simulink library "Differential_Gear1DShafts3Dfix"  (R2026a)
settings: Solver=VariableStepAuto
undefined symbols (not defined in the file): Shaft1D, Shaft3D, X, Y, Z
libraries: sm_lib x5, Differential_Components x2, fl_lib x2, nesl_utility x2, sdl_lib x1
Description:
  | Component of Simscape Vehicle Templates Library
  | 
  | Copyright 2018-2026 The MathWorks, Inc.
settings Model: Creator=smiller  LastModifiedBy=smiller

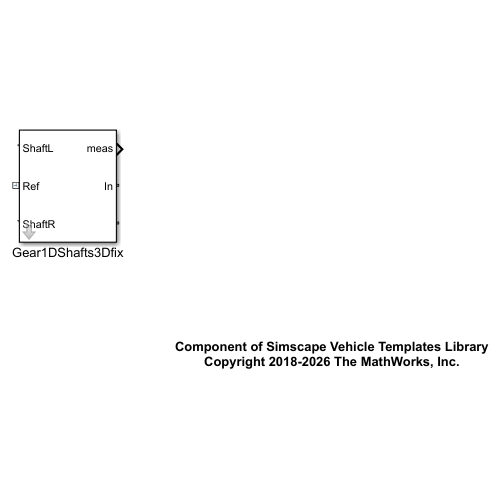
[thumbnail: Simulink's stored preview of the top-level diagram]
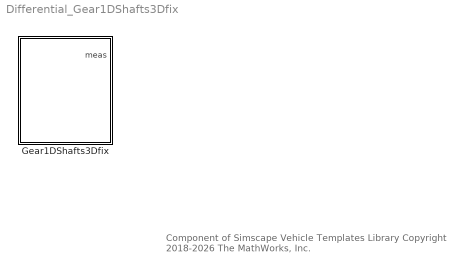
== system Differential_Gear1DShafts3Dfix ==
  note: Component of Simscape Vehicle Templates Library
      | Copyright 2018-2026 The MathWorks, Inc.
  Gear1DShafts3Dfix : Subsystem  VariantControl=Gear1DShafts3Dfix  mask(Differential 1D with static 3D Shafts){}
      mask help: Differential power transmission using 1D mechanical model. 3D shafts do not rotate and are included for 3D visualization and to contribute nonrotating mass and inertia.

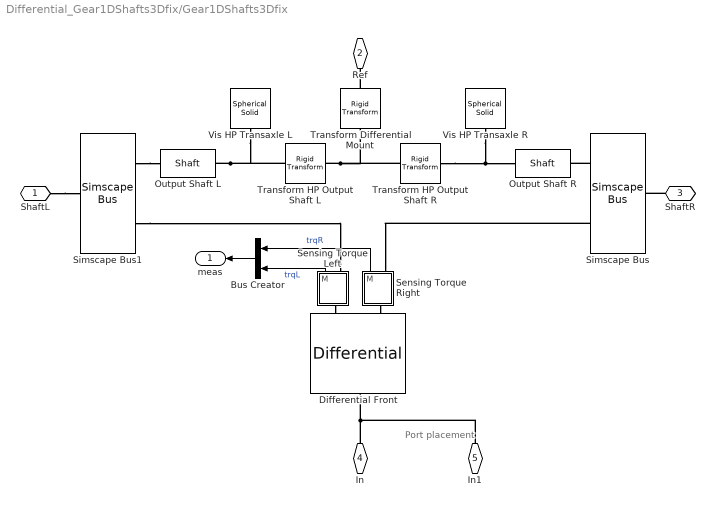
== system Differential_Gear1DShafts3Dfix/Gear1DShafts3Dfix ==
  note: Port
      | placement
  Bus Creator : BusCreator  Inputs=2
  Differential Front : sdl_lib/Gears/Differential  driveshaft_location=2  cd_ratio=Differential.ratio.Value  friction_model=1  efficiency=[.85, .92]  temperature_TLU=[280, 300, 320] K  efficiency_ss_TLU=[.95, .9, .85]  efficiency_cd_TLU=[.95, .9, .85]  pwr_thr=[.001, .001] W  mu_visc=[0, 0] N*m/(rad/s)  model_inertia=0  sun_inertia=1e-10 kg*m^2  sun_radius=0.01 m  carrier_inertia=0.001 kg*m^2  planet_inertia=0.001 kg*m^2  planet_mass=1e-10 kg  thermal_mass=50 J/K  T_init=300 K
  Output Shaft L : Differential_Components/Shaft  popup_leftRight=Left  shaft_m=Differential.ShaftOutL.m.Value  len_shaft=Differential.ShaftOutL.l.Value  clr_shaft=Visual.DiffShaftOut.clr  opc_shaft=Visual.part.opc  rad_shaft=Visual.DiffShaftOut.rad
  Output Shaft R : Differential_Components/Shaft  popup_leftRight=Right  shaft_m=Differential.ShaftOutR.m.Value  len_shaft=Differential.ShaftOutR.l.Value  clr_shaft=Visual.DiffShaftOut.clr  opc_shaft=Visual.part.opc  rad_shaft=Visual.DiffShaftOut.rad
  Sensing Torque Left : Subsystem
  Sensing Torque Right : Subsystem
  Simscape Bus : SimscapeBus  HierarchyStrings=Shaft3D;Shaft1D
  Simscape Bus1 : SimscapeBus  HierarchyStrings=Shaft3D;Shaft1D
  Transform Differential Mount : sm_lib/Frames and Transforms/Rigid Transform  RotationMethod=None  FollAlignAxisA=+X  BaseAlignAxisA=+Y  FollAlignAxisB=+Y  BaseAlignAxisB=+Z  RotationStandardAxis=+Z  RotationAngle=0.0  RotationAngleUnits=deg  RotationArbitraryAxis=[0 0 1]  RotationSequenceAxes=FollowerAxes  RotationSequence=XYX  RotationSequenceAngles=[0 0 0]  RotationSequenceAnglesUnits=deg  RotationMatrix=[1 0 0; 0 1 0; 0 0 1]  Quaternion=[1 0 0 0]  TranslationMethod=Cartesian  TranslationCartesianOffset=Differential.sMount.Value  TranslationCartesianOffsetUnits=m  TranslationStandardAxis=+Z  TranslationStandardOffset=0  TranslationStandardOffsetUnits=m  TranslationROffset=0  TranslationROffsetUnits=m  TranslationThetaOffset=0  TranslationThetaOffsetUnits=deg  TranslationZOffset=0  TranslationZOffsetUnits=m
  Transform HP Output Shaft L : sm_lib/Frames and Transforms/Rigid Transform  RotationMethod=StandardAxis  FollAlignAxisA=+X  BaseAlignAxisA=+Y  FollAlignAxisB=+Y  BaseAlignAxisB=+Z  RotationStandardAxis=+X  RotationAngle=-90  RotationAngleUnits=deg  RotationArbitraryAxis=[0 0 1]  RotationSequenceAxes=FollowerAxes  RotationSequence=XYX  RotationSequenceAngles=[0 0 0]  RotationSequenceAnglesUnits=deg  RotationMatrix=[1 0 0; 0 1 0; 0 0 1]  Quaternion=[1 0 0 0]  TranslationMethod=Cartesian  TranslationCartesianOffset=Differential.ShaftOutL.sInboard.Value  TranslationCartesianOffsetUnits=m  TranslationStandardAxis=+Z  TranslationStandardOffset=0  TranslationStandardOffsetUnits=m  TranslationROffset=0  TranslationROffsetUnits=m  TranslationThetaOffset=0  TranslationThetaOffsetUnits=deg  TranslationZOffset=0  TranslationZOffsetUnits=m
  Transform HP Output Shaft R : sm_lib/Frames and Transforms/Rigid Transform  RotationMethod=StandardAxis  FollAlignAxisA=+X  BaseAlignAxisA=+Y  FollAlignAxisB=+Y  BaseAlignAxisB=+Z  RotationStandardAxis=+X  RotationAngle=-90  RotationAngleUnits=deg  RotationArbitraryAxis=[0 0 1]  RotationSequenceAxes=FollowerAxes  RotationSequence=XYX  RotationSequenceAngles=[0 0 0]  RotationSequenceAnglesUnits=deg  RotationMatrix=[1 0 0; 0 1 0; 0 0 1]  Quaternion=[1 0 0 0]  TranslationMethod=Cartesian  TranslationCartesianOffset=Differential.ShaftOutR.sInboard.Value  TranslationCartesianOffsetUnits=m  TranslationStandardAxis=+Z  TranslationStandardOffset=0  TranslationStandardOffsetUnits=m  TranslationROffset=0  TranslationROffsetUnits=m  TranslationThetaOffset=0  TranslationThetaOffsetUnits=deg  TranslationZOffset=0  TranslationZOffsetUnits=m
  Vis HP Transaxle L : sm_lib/Body Elements/Spherical Solid  SphereRadius=Visual.hp.rad  SphereRadiusUnits=m  ExportEntireGeometry=off  InertiaType=CalculateFromGeometry  BasedOnType=Density  Density=0  DensityUnits=kg/m^3  Mass=1  MassUnits=kg  CenterOfMass=[0 0 0]  CenterOfMassUnits=m  MomentsOfInertia=[1 1 1]  MomentsOfInertiaUnits=kg*m^2  ProductsOfInertia=[0 0 0]  ProductsOfInertiaUnits=kg*m^2  GraphicType=FromGeometry  MarkerShape=Sphere  MarkerSize=10  GraphicVisPropType=SimpleVisualProperties  GraphicDiffuseColor=Visual.hp.clr  GraphicOpacity=Visual.hp.opc  GraphicSpecularColor=[0.5 0.5 0.5 1.0]  GraphicAmbientColor=[0.15 0.15 0.15 1.0]  GraphicEmissiveColor=[0.0 0.0 0.0 1.0]  GraphicShininess=75  DoExposeReferenceFrame=on  SerializedFrames=<Frames/>
  Vis HP Transaxle R : sm_lib/Body Elements/Spherical Solid  SphereRadius=Visual.hp.rad  SphereRadiusUnits=m  ExportEntireGeometry=off  InertiaType=CalculateFromGeometry  BasedOnType=Density  Density=0  DensityUnits=kg/m^3  Mass=1  MassUnits=kg  CenterOfMass=[0 0 0]  CenterOfMassUnits=m  MomentsOfInertia=[1 1 1]  MomentsOfInertiaUnits=kg*m^2  ProductsOfInertia=[0 0 0]  ProductsOfInertiaUnits=kg*m^2  GraphicType=FromGeometry  MarkerShape=Sphere  MarkerSize=10  GraphicVisPropType=SimpleVisualProperties  GraphicDiffuseColor=Visual.hp.clr  GraphicOpacity=Visual.hp.opc  GraphicSpecularColor=[0.5 0.5 0.5 1.0]  GraphicAmbientColor=[0.15 0.15 0.15 1.0]  GraphicEmissiveColor=[0.0 0.0 0.0 1.0]  GraphicShininess=75  DoExposeReferenceFrame=on  SerializedFrames=<Frames/>
  ShaftL : PMIOPort  Side=Left
  Ref : PMIOPort  Port=2  Side=Left
  ShaftR : PMIOPort  Port=3  Side=Left
  In : PMIOPort  Port=4  Side=Right
  In1 : PMIOPort  Port=5  Side=Right
  meas : Outport  VectorParamsAs1DForOutWhenUnconnected=off
  wires:
  Sensing Torque Right/1(M) -> Bus Creator/1  "trqR"
  Sensing Torque Left/1(M) -> Bus Creator/2  "trqL"
  Bus Creator/1 -> meas/1
  connections:
  Sensing Torque Right/LConn1 -- Differential Front/RConn1
  Sensing Torque Left/LConn1 -- Differential Front/RConn2
  Simscape Bus1/LConn1 -- Output Shaft L/LConn1
  ShaftL/RConn1 -- Simscape Bus1/RConn1
  ShaftR/RConn1 -- Simscape Bus/RConn1
  Simscape Bus1/LConn2 -- Sensing Torque Left/RConn1
  Transform Differential Mount/LConn1 -- Ref/RConn1
  Simscape Bus/LConn2 -- Sensing Torque Right/RConn1
  Simscape Bus/LConn1 -- Output Shaft R/LConn1
  Transform HP Output Shaft R/RConn1 -- Output Shaft R/RConn1 -- Vis HP Transaxle R/RConn1
  Transform HP Output Shaft L/LConn1 -- Transform Differential Mount/RConn1 -- Transform HP Output Shaft R/LConn1
  Output Shaft L/RConn1 -- Transform HP Output Shaft L/RConn1 -- Vis HP Transaxle L/RConn1
  In/RConn1 -- Differential Front/LConn1 -- In1/RConn1

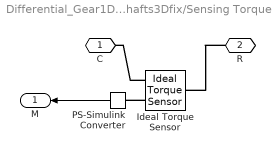
== system Differential_Gear1DShafts3Dfix/Gear1DShafts3Dfix/Sensing Torque Left ==
  Ideal Torque Sensor : fl_lib/Mechanical/Mechanical Sensors/Ideal Torque Sensor
  PS-Simulink Converter : nesl_utility/PS-Simulink Converter  PhysicalDomain=network_engine_domain  SubClassName=ps_output  LeftPortType=input  RightPortType=output  PseudoPeriodic=off  Frequencies=[]  VectorFormat=1-D array  Unit=N*m  AffineConversion=off
  C : PMIOPort  Side=Right
  R : PMIOPort  Port=2  Side=Left
  M : Outport  VectorParamsAs1DForOutWhenUnconnected=off
  wires:
  PS-Simulink Converter/1 -> M/1
  connections:
  Ideal Torque Sensor/RConn2 -- PS-Simulink Converter/LConn1
  R/RConn1 -- Ideal Torque Sensor/LConn1
  Ideal Torque Sensor/RConn1 -- C/RConn1

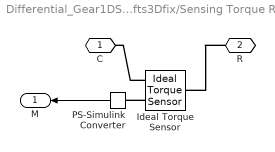
== system Differential_Gear1DShafts3Dfix/Gear1DShafts3Dfix/Sensing Torque Right ==
  Ideal Torque Sensor : fl_lib/Mechanical/Mechanical Sensors/Ideal Torque Sensor
  PS-Simulink Converter : nesl_utility/PS-Simulink Converter  PhysicalDomain=network_engine_domain  SubClassName=ps_output  LeftPortType=input  RightPortType=output  PseudoPeriodic=off  Frequencies=[]  VectorFormat=1-D array  Unit=N*m  AffineConversion=off
  C : PMIOPort  Side=Right
  R : PMIOPort  Port=2  Side=Left
  M : Outport  VectorParamsAs1DForOutWhenUnconnected=off
  wires:
  PS-Simulink Converter/1 -> M/1
  connections:
  Ideal Torque Sensor/RConn1 -- C/RConn1
  R/RConn1 -- Ideal Torque Sensor/LConn1
  Ideal Torque Sensor/RConn2 -- PS-Simulink Converter/LConn1
